simulink model "lagging_compensator_simulink"  (R2016a)
settings: Solver=VariableStepAuto  StartTime=0.0  StopTime=100  RelTol=1e-3
values from neighbouring files (symbols this model uses):
  Kc = Kp_desejado/Kp_antigo    (= 99)    [adv_lag_igual.m]    (also in advance_and_lagging_compensator.m = (1)/abs(((s1+zero_adv)/(s1+polo_adv))*planta); advance_compensator.m = (1)/abs(((s1+zero_cont1)/(s1+polo_cont1))*planta); lagging_compensator.m = (1)/abs(((s1+zero_lag)/(s1+polo_lag))*planta))
  polo_lag = 1/(beta*T2)    (= 0.0702229578913)    [adv_lag_igual.m]    (also in advance_and_lagging_compensator.m = 1/(beta*T2); lagging_compensator.m = 1/(beta*T))
  zero_lag = 0.7    [adv_lag_igual.m]    (also in advance_and_lagging_compensator.m = input('Escolha um Zero para o controlador perto da Origem-> ; lagging_compensator.m = input('Escolha um Zero para o controlador PERTO DE ZERO-> '))
settings Model: Creator=jessa  LastModifiedBy=jessa

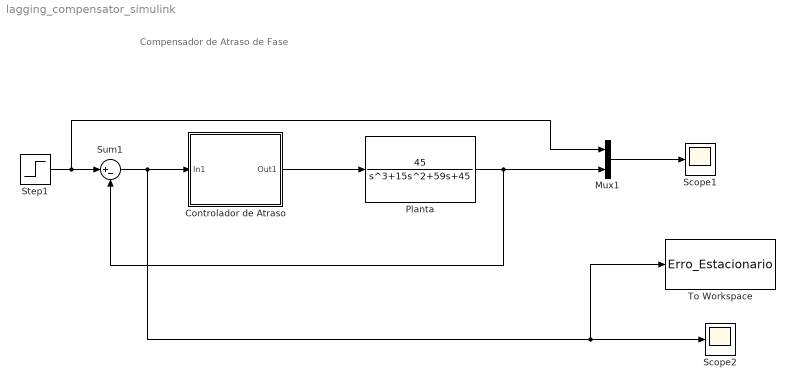
== system lagging_compensator_simulink ==
  note: Compensador de Atraso de Fase
  Controlador de Atraso : Subsystem
  Mux1 : Mux  Inputs=2
  Planta : TransferFcn  Numerator=[45]  Denominator=[1 15 59 45]
  Scope1 : Scope
  Scope2 : Scope
  Step1 : Step  Time=0  SampleTime=0
  Sum1 : Sum  Inputs=|+-
  To Workspace : ToWorkspace  VariableName=Erro_Estacionario  SampleTime=-1
  wires:
  Mux1/1 -> Scope1/1
  Planta/1 -> Sum1/2, Mux1/2
  Step1/1 -> Sum1/1, Mux1/1
  Sum1/1 -> To Workspace/1, Scope2/1, Controlador de Atraso/1(In1)
  Controlador de Atraso/1(Out1) -> Planta/1

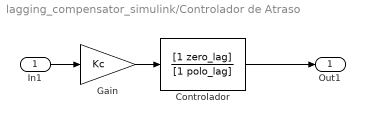
== system lagging_compensator_simulink/Controlador de Atraso ==
  In1 : Inport
  Controlador : TransferFcn  Numerator=[1 zero_lag]  Denominator=[1 polo_lag]
  Gain : Gain  Gain=Kc
  Out1 : Outport
  wires:
  In1/1 -> Gain/1
  Gain/1 -> Controlador/1
  Controlador/1 -> Out1/1
